simulink subsystem "API221_Wash"  (R2022b)
settings: Solver=VariableStepAuto  StartTime=0.0  StopTime=10.0  RelTol=1e-3
settings Model: Creator=PROSTJP  LastModifiedBy=PAVULV

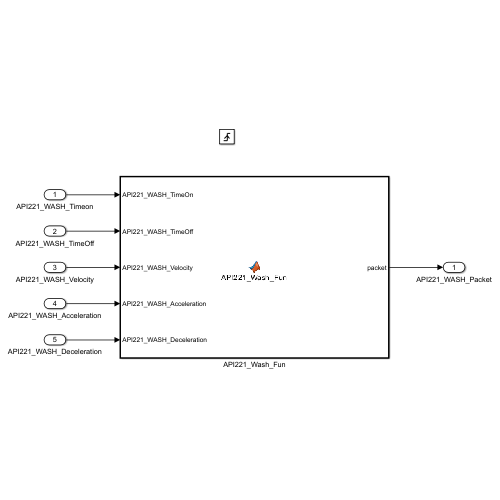
[thumbnail: Simulink's stored preview of the top-level diagram]
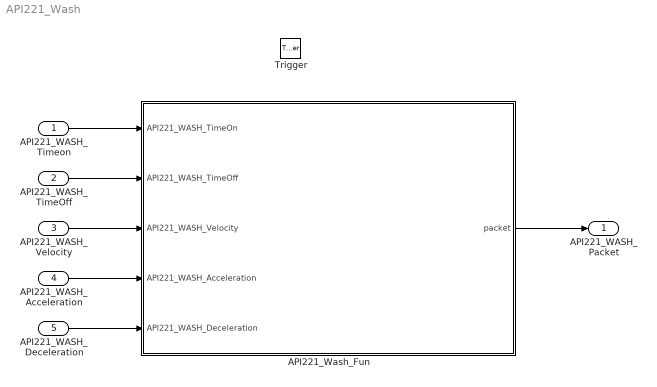
== system API221_Wash ==
  API221_WASH_Timeon : Inport
  API221_WASH_TimeOff : Inport  Port=2
  API221_WASH_Velocity : Inport  Port=3
  API221_WASH_Acceleration : Inport  Port=4
  API221_WASH_Deceleration : Inport  Port=5
  Trigger : TriggerPort  VariantControl=(inherit)  PortDimensions=1
  API221_Wash_Fun : MATLAB Function  TreatAsAtomicUnit=on
  API221_WASH_Packet : Outport
  wires:
  API221_Wash_Fun/1(packet) -> API221_WASH_Packet/1
  API221_WASH_Acceleration/1 -> API221_Wash_Fun/4(API221_WASH_Acceleration)
  API221_WASH_Velocity/1 -> API221_Wash_Fun/3(API221_WASH_Velocity)
  API221_WASH_Timeon/1 -> API221_Wash_Fun/1(API221_WASH_TimeOn)
  API221_WASH_TimeOff/1 -> API221_Wash_Fun/2(API221_WASH_TimeOff)
  API221_WASH_Deceleration/1 -> API221_Wash_Fun/5(API221_WASH_Deceleration)

== matlab function API221_Wash/API221_Wash_Fun ==
  data: packet output uint8 [1..100]; API221_WASH_TimeOn input; API221_WASH_TimeOff input; API221_WASH_Velocity input; API221_WASH_Acceleration input; API221_WASH_Deceleration input
function packet = API221_Wash_Fun(API221_WASH_TimeOn, API221_WASH_TimeOff, API221_WASH_Velocity, API221_WASH_Acceleration, API221_WASH_Deceleration)

     
    crc_dummy = 0; % Crc check on win packet not implemented
    PAD_SIZE = 100; 
    %sim_stop_time = 180;
    % API 221  - PULSE
    % HEADER
    destination = 0;
    node_id = 1;
    sdu_length = 13;
    sap = 4;
    api_id = 221;
    op_code = 13;
    cmd_fb = 0;
    frag = 0;
    mmp = 0;
    destination_source = destination + node_id * (2^4);
    opcode_compl = op_code + cmd_fb * (2^5) + frag * (2^6) + mmp * (2^7);

    motor_idx = uint8(0);
    
    header_api221 = uint8([destination_source sap sdu_length api_id opcode_compl]);
    
    packet = zeros(PAD_SIZE,1,'uint8');
    
    t_on_arr  = uint8([bitshift(API221_WASH_TimeOn,-8), bitand(API221_WASH_TimeOn,0x00FF)]);
    t_off_arr = uint8([bitshift(API221_WASH_TimeOff,-8), bitand(API221_WASH_TimeOff,0x00FF)]);
    speed_arr = uint8([bitshift(API221_WASH_Velocity,-8), bitand(API221_WASH_Velocity,0x00FF)]);
    accel_arr = uint8([bitshift(API221_WASH_Acceleration,-8), bitand(API221_WASH_Acceleration,0x00FF)]);
    decel_arr = uint8([bitshift(API221_WASH_Deceleration,-8), bitand(API221_WASH_Deceleration,0x00FF)]);        

    tmp = uint8([header_api221 motor_idx t_on_arr t_off_arr speed_arr accel_arr decel_arr crc_dummy]);
    packet(1:length(tmp)) = tmp(:);
